simulink model "example"  (Simulink 6.1)
settings: Solver=ode45  StartTime=0.0  StopTime=5  RelTol=1e-3
settings Model: LastModifiedBy=Charles
settings DataIOCC: LimitDataPoints=off  SaveOutput=off  SaveTime=off
settings OptimizationCC: InlineParams=on  InlineInvariantSignals=off
settings DebuggingCC: SignalResolutionControl=UseLocalSettings
settings HardwareCC: TargetUnknown=on
settings GRTTargetCC: ModelReferenceCompliant=off  MatFileLogging=off

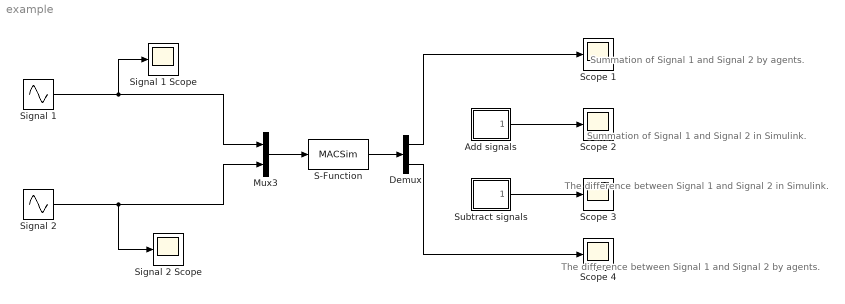
== system example ==
  note: Summation of
      | Signal 1 and Signal 2
      | by agents.
  note: The difference between
      | Signal 1 and Signal 2
      | by agents.
  note: Summation of
      | Signal 1 and Signal 2
      | in Simulink.
  note: The difference between
      | Signal 1 and Signal 2
      | in Simulink.
  Add signals : Subsystem
  Demux : Demux  Outputs=2
  Mux3 : Mux  Inputs=2
  S-Function : S-Function  FunctionName=MACSim
  Scope {1..4} (4 alike) : Scope
      Scope 2 settings: SaveName=ScopeData2
      Scope 3 settings: SaveName=ScopeData3
  Signal 1 : Sin  Frequency=2  Phase=3.14159  SampleTime=0
  Signal 1 Scope : Scope
      settings: SaveName=ScopeData4
  Signal 2 : Sin  Amplitude=2  SampleTime=0
  Signal 2 Scope : Scope
      settings: SaveName=ScopeData5
  Subtract signals : Subsystem
  wires:
  Mux3/1 -> S-Function/1
  S-Function/1 -> Demux/1
  Demux/1 -> Scope 1/1
  Demux/2 -> Scope 4/1
  Signal 1/1 -> Signal 1 Scope/1, Mux3/1
  Signal 2/1 -> Signal 2 Scope/1, Mux3/2
  Add signals/1(Out1) -> Scope 2/1
  Subtract signals/1(Out1) -> Scope 3/1

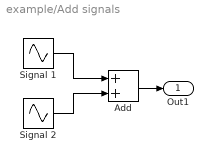
== system example/Add signals ==
  Add : Sum  OutScaling=2^-10
  Signal 1 : Sin  Frequency=2  Phase=3.14159  SampleTime=0
  Signal 2 : Sin  Amplitude=2  SampleTime=0
  Out1 : Outport
  wires:
  Signal 1/1 -> Add/1
  Signal 2/1 -> Add/2
  Add/1 -> Out1/1

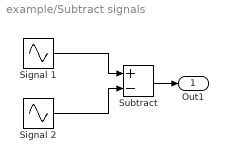
== system example/Subtract signals ==
  Signal 1 : Sin  Frequency=2  Phase=3.14159  SampleTime=0
  Signal 2 : Sin  Amplitude=2  SampleTime=0
  Subtract : Sum  Inputs=+-  OutScaling=2^-10
  Out1 : Outport
  wires:
  Signal 1/1 -> Subtract/1
  Signal 2/1 -> Subtract/2
  Subtract/1 -> Out1/1
